simulink model "sus"  (Simulink 6.5)
settings: Solver=ode45  StartTime=0.0  StopTime=16  RelTol=1e-3
libraries: cdsFilt x266, cdsBitwise x92, cdsEpicsOut x84, cdsEpicsBinIn x56, cdsEpicsIn x20, cdsFiltCtrl x18, cdsMatrix x11, cdsSwitch x7, cdsWD x7, cdsFunctionCall x5, cdsRio1 x4, dac x3
(part 2 of 20)

== system sus/LOCK ==
  note: All Outputs the same
  In5 : Inport
  In6 : Inport  Port=2
  In7 : Inport  Port=3
  In8 : Inport  Port=4
  CODE : cdsFunctionCall/Subsystem  Tag=cdsFunctionCall  Description=|  SystemSampleTime=-1
      | Allows to make a call to external C function from the front-end code.                                            
      | User needs to use a Mux and a Demux to proved N number of inputs and M number of outputs to an external function.
      | Function "Foo()" code needs to be put in a file Foo.c in advLigo/src/fe/<model> directory.
      settings: AttributesFormatString=%<Tag>
  DIG4 : cdsFilt/Subsystem  Tag=cdsFilt  Description=|  SystemSampleTime=-1
      | Purpose:                                                                                                                                                                                                                                  
      | Standard CDS IIR filter module.                                                                                                                                                                                                           
      |                                                                                                                                                                                                                                           
      | Operation:                                                                                                                                                                                                                                
      | Consists of 10 second order section IIR filters, plus a ramped gain stage. In FE code, also provides pre-defined test points and excitation channel inputs. The filter coefficients are defined in the LIGO system using the 'foton' tool.
      |                                                                                                                                                                                                                                           
      | Usage:                                                                                                                                                                                                                                    
      | Name the part with the desired filter module name.
      settings: AttributesFormatString=%<Tag>
  Demux : Demux  Outputs=5
  Ground1 : Ground
  Ground7 : Ground
  Mux : Mux  Inputs=6
  OFF : cdsEpicsIn/Subsystem  Tag=cdsEpicsInput  Description=|  SystemSampleTime=-1
      | Purpose:                                                                              
      | Create an EPICS input channel connection to the FE realtime controls.                 
      |                                                                                       
      | Operation:                                                                            
      | Outputs value from an EPICS ai record. Value is floating point with a precision of 3..
      |                                                                                       
      | Usage:                                                                                
      | Name the part with the desired EPICS channel name.
      settings: AttributesFormatString=%<Tag>
  ON : cdsEpicsIn/Subsystem  Tag=cdsEpicsInput  Description=|  SystemSampleTime=-1
      | Purpose:                                                                              
      | Create an EPICS input channel connection to the FE realtime controls.                 
      |                                                                                       
      | Operation:                                                                            
      | Outputs value from an EPICS ai record. Value is floating point with a precision of 3..
      |                                                                                       
      | Usage:                                                                                
      | Name the part with the desired EPICS channel name.
      settings: AttributesFormatString=%<Tag>
  REFL_DC : cdsFilt/Subsystem  Tag=cdsFilt  Description=|  SystemSampleTime=-1
      | Purpose:                                                                                                                                                                                                                                  
      | Standard CDS IIR filter module.                                                                                                                                                                                                           
      |                                                                                                                                                                                                                                           
      | Operation:                                                                                                                                                                                                                                
      | Consists of 10 second order section IIR filters, plus a ramped gain stage. In FE code, also provides pre-defined test points and excitation channel inputs. The filter coefficients are defined in the LIGO system using the 'foton' tool.
      |                                                                                                                                                                                                                                           
      | Usage:                                                                                                                                                                                                                                    
      | Name the part with the desired filter module name.
      settings: AttributesFormatString=%<Tag>
  REFL_I : cdsFilt/Subsystem  Tag=cdsFilt  Description=|  SystemSampleTime=-1
      | Purpose:                                                                                                                                                                                                                                  
      | Standard CDS IIR filter module.                                                                                                                                                                                                           
      |                                                                                                                                                                                                                                           
      | Operation:                                                                                                                                                                                                                                
      | Consists of 10 second order section IIR filters, plus a ramped gain stage. In FE code, also provides pre-defined test points and excitation channel inputs. The filter coefficients are defined in the LIGO system using the 'foton' tool.
      |                                                                                                                                                                                                                                           
      | Usage:                                                                                                                                                                                                                                    
      | Name the part with the desired filter module name.
      settings: AttributesFormatString=%<Tag>
  TRAN_DC : cdsFilt/Subsystem  Tag=cdsFilt  Description=|  SystemSampleTime=-1
      | Purpose:                                                                                                                                                                                                                                  
      | Standard CDS IIR filter module.                                                                                                                                                                                                           
      |                                                                                                                                                                                                                                           
      | Operation:                                                                                                                                                                                                                                
      | Consists of 10 second order section IIR filters, plus a ramped gain stage. In FE code, also provides pre-defined test points and excitation channel inputs. The filter coefficients are defined in the LIGO system using the 'foton' tool.
      |                                                                                                                                                                                                                                           
      | Usage:                                                                                                                                                                                                                                    
      | Name the part with the desired filter module name.
      settings: AttributesFormatString=%<Tag>
  Out1 : Outport
  Out2 : Outport  Port=2
  Out3 : Outport  Port=3
  Out4 : Outport  Port=4
  Out5 : Outport  Port=5
  wires:
  CODE/1 -> Demux/1
  Mux/1 -> CODE/1
  Demux/1 -> Out1/1
  Demux/2 -> Out2/1
  Demux/3 -> Out3/1
  Demux/4 -> Out4/1
  Demux/5 -> Out5/1
  In5/1 -> REFL_I/1
  REFL_I/1 -> Mux/1
  TRAN_DC/1 -> Mux/2
  In6/1 -> TRAN_DC/1
  In7/1 -> REFL_DC/1
  REFL_DC/1 -> Mux/3
  In8/1 -> DIG4/1
  DIG4/1 -> Mux/4
  ON/1 -> Mux/5
  OFF/1 -> Mux/6
  Ground7/1 -> ON/1
  Ground1/1 -> OFF/1

== system sus/MON_M0 ==
  NoiseF1 : Inport  OutDataType=fixdt(1,16,0)  OutScaling=[]
  VoltF1 : Inport  Port=2  OutDataType=fixdt(1,16,0)  OutScaling=[]
  FastF1 : Inport  Port=3  OutDataType=fixdt(1,16,0)  OutScaling=[]
  SlowF1 : Inport  Port=4  OutDataType=fixdt(1,16,0)  OutScaling=[]
  NoiseF2 : Inport  Port=5  OutDataType=fixdt(1,16,0)  OutScaling=[]
  VoltF2 : Inport  Port=6  OutDataType=fixdt(1,16,0)  OutScaling=[]
  FastF2 : Inport  Port=7  OutDataType=fixdt(1,16,0)  OutScaling=[]
  SlowF2 : Inport  Port=8  OutDataType=fixdt(1,16,0)  OutScaling=[]
  NoiseF3 : Inport  Port=9  OutDataType=fixdt(1,16,0)  OutScaling=[]
  VoltF3 : Inport  Port=10  OutDataType=fixdt(1,16,0)  OutScaling=[]
  FastF3 : Inport  Port=11  OutDataType=fixdt(1,16,0)  OutScaling=[]
  SlowF3 : Inport  Port=12  OutDataType=fixdt(1,16,0)  OutScaling=[]
  NoiseLeft : Inport  Port=13  OutDataType=fixdt(1,16,0)  OutScaling=[]
  VoltLeft : Inport  Port=14  OutDataType=fixdt(1,16,0)  OutScaling=[]
  FastLeft : Inport  Port=15  OutDataType=fixdt(1,16,0)  OutScaling=[]
  SlowLeft : Inport  Port=16  OutDataType=fixdt(1,16,0)  OutScaling=[]
  NoiseRight : Inport  Port=17  OutDataType=fixdt(1,16,0)  OutScaling=[]
  VoltRight : Inport  Port=18  OutDataType=fixdt(1,16,0)  OutScaling=[]
  FastRight : Inport  Port=19  OutDataType=fixdt(1,16,0)  OutScaling=[]
  SlowRight : Inport  Port=20  OutDataType=fixdt(1,16,0)  OutScaling=[]
  NoiseSide : Inport  Port=21  OutDataType=fixdt(1,16,0)  OutScaling=[]
  VoltSide : Inport  Port=22  OutDataType=fixdt(1,16,0)  OutScaling=[]
  FastSide : Inport  Port=23  OutDataType=fixdt(1,16,0)  OutScaling=[]
  SlowSide : Inport  Port=24  OutDataType=fixdt(1,16,0)  OutScaling=[]
  FACE1 : Subsystem
  FACE2 : Subsystem
  FACE3 : Subsystem
  LEFT : Subsystem
  RIGHT : Subsystem
  SIDE : Subsystem
  wires:
  NoiseF1/1 -> FACE1/1(Noise)
  VoltF1/1 -> FACE1/2(Volt)
  FastF1/1 -> FACE1/3(Fast I)
  SlowF1/1 -> FACE1/4(Slow I)
  NoiseF2/1 -> FACE2/1(Noise)
  VoltF2/1 -> FACE2/2(Volt)
  FastF2/1 -> FACE2/3(Fast I)
  SlowF2/1 -> FACE2/4(Slow I)
  NoiseF3/1 -> FACE3/1(Noise)
  VoltF3/1 -> FACE3/2(Volt)
  FastF3/1 -> FACE3/3(Fast I)
  SlowF3/1 -> FACE3/4(Slow I)
  NoiseLeft/1 -> LEFT/1(Noise)
  VoltLeft/1 -> LEFT/2(Volt)
  FastLeft/1 -> LEFT/3(Fast I)
  SlowLeft/1 -> LEFT/4(Slow I)
  NoiseRight/1 -> RIGHT/1(Noise)
  VoltRight/1 -> RIGHT/2(Volt)
  FastRight/1 -> RIGHT/3(Fast I)
  SlowRight/1 -> RIGHT/4(Slow I)
  NoiseSide/1 -> SIDE/1(Noise)
  VoltSide/1 -> SIDE/2(Volt)
  FastSide/1 -> SIDE/3(Fast I)
  SlowSide/1 -> SIDE/4(Slow I)

== system sus/MON_PEN ==
  NoiseUL : Inport  OutDataType=fixdt(1,16,0)  OutScaling=[]
  VoltUL : Inport  Port=2  OutDataType=fixdt(1,16,0)  OutScaling=[]
  FastUL : Inport  Port=3  OutDataType=fixdt(1,16,0)  OutScaling=[]
  SlowUL : Inport  Port=4  OutDataType=fixdt(1,16,0)  OutScaling=[]
  NoiseLL : Inport  Port=5  OutDataType=fixdt(1,16,0)  OutScaling=[]
  VoltLL : Inport  Port=6  OutDataType=fixdt(1,16,0)  OutScaling=[]
  FastLL : Inport  Port=7  OutDataType=fixdt(1,16,0)  OutScaling=[]
  SlowLL : Inport  Port=8  OutDataType=fixdt(1,16,0)  OutScaling=[]
  NoiseUR : Inport  Port=9  OutDataType=fixdt(1,16,0)  OutScaling=[]
  VoltUR : Inport  Port=10  OutDataType=fixdt(1,16,0)  OutScaling=[]
  FastUR : Inport  Port=11  OutDataType=fixdt(1,16,0)  OutScaling=[]
  SlowUR : Inport  Port=12  OutDataType=fixdt(1,16,0)  OutScaling=[]
  NoiseLR : Inport  Port=13  OutDataType=fixdt(1,16,0)  OutScaling=[]
  VoltLR : Inport  Port=14  OutDataType=fixdt(1,16,0)  OutScaling=[]
  FastLR : Inport  Port=15  OutDataType=fixdt(1,16,0)  OutScaling=[]
  SlowLR : Inport  Port=16  OutDataType=fixdt(1,16,0)  OutScaling=[]
  LL : Subsystem
  LR : Subsystem
  UL : Subsystem
  UR : Subsystem
  wires:
  NoiseUL/1 -> UL/1(Noise)
  VoltUL/1 -> UL/2(Volt)
  FastUL/1 -> UL/3(Fast I)
  SlowUL/1 -> UL/4(Slow I)
  NoiseLL/1 -> LL/1(Noise)
  VoltLL/1 -> LL/2(Volt)
  FastLL/1 -> LL/3(Fast I)
  SlowLL/1 -> LL/4(Slow I)
  NoiseUR/1 -> UR/1(Noise)
  VoltUR/1 -> UR/2(Volt)
  FastUR/1 -> UR/3(Fast I)
  SlowUR/1 -> UR/4(Slow I)
  NoiseLR/1 -> LR/1(Noise)
  VoltLR/1 -> LR/2(Volt)
  FastLR/1 -> LR/3(Fast I)
  SlowLR/1 -> LR/4(Slow I)

== system sus/MON_R0 ==
  NoiseF1 : Inport  OutDataType=fixdt(1,16,0)  OutScaling=[]
  VoltF1 : Inport  Port=2  OutDataType=fixdt(1,16,0)  OutScaling=[]
  FastF1 : Inport  Port=3  OutDataType=fixdt(1,16,0)  OutScaling=[]
  SlowF1 : Inport  Port=4  OutDataType=fixdt(1,16,0)  OutScaling=[]
  NoiseF2 : Inport  Port=5  OutDataType=fixdt(1,16,0)  OutScaling=[]
  VoltF2 : Inport  Port=6  OutDataType=fixdt(1,16,0)  OutScaling=[]
  FastF2 : Inport  Port=7  OutDataType=fixdt(1,16,0)  OutScaling=[]
  SlowF2 : Inport  Port=8  OutDataType=fixdt(1,16,0)  OutScaling=[]
  NoiseF3 : Inport  Port=9  OutDataType=fixdt(1,16,0)  OutScaling=[]
  VoltF3 : Inport  Port=10  OutDataType=fixdt(1,16,0)  OutScaling=[]
  FastF3 : Inport  Port=11  OutDataType=fixdt(1,16,0)  OutScaling=[]
  SlowF3 : Inport  Port=12  OutDataType=fixdt(1,16,0)  OutScaling=[]
  NoiseLeft : Inport  Port=13  OutDataType=fixdt(1,16,0)  OutScaling=[]
  VoltLeft : Inport  Port=14  OutDataType=fixdt(1,16,0)  OutScaling=[]
  FastLeft : Inport  Port=15  OutDataType=fixdt(1,16,0)  OutScaling=[]
  SlowLeft : Inport  Port=16  OutDataType=fixdt(1,16,0)  OutScaling=[]
  NoiseRight : Inport  Port=17  OutDataType=fixdt(1,16,0)  OutScaling=[]
  VoltRight : Inport  Port=18  OutDataType=fixdt(1,16,0)  OutScaling=[]
  FastRight : Inport  Port=19  OutDataType=fixdt(1,16,0)  OutScaling=[]
  SlowRight : Inport  Port=20  OutDataType=fixdt(1,16,0)  OutScaling=[]
  NoiseSide : Inport  Port=21  OutDataType=fixdt(1,16,0)  OutScaling=[]
  VoltSide : Inport  Port=22  OutDataType=fixdt(1,16,0)  OutScaling=[]
  FastSide : Inport  Port=23  OutDataType=fixdt(1,16,0)  OutScaling=[]
  SlowSide : Inport  Port=24  OutDataType=fixdt(1,16,0)  OutScaling=[]
  FACE1 : Subsystem
  FACE2 : Subsystem
  FACE3 : Subsystem
  LEFT : Subsystem
  RIGHT : Subsystem
  SIDE : Subsystem
  wires:
  NoiseF1/1 -> FACE1/1(Noise)
  VoltF1/1 -> FACE1/2(Volt)
  FastF1/1 -> FACE1/3(Fast I)
  SlowF1/1 -> FACE1/4(Slow I)
  NoiseF2/1 -> FACE2/1(Noise)
  VoltF2/1 -> FACE2/2(Volt)
  FastF2/1 -> FACE2/3(Fast I)
  SlowF2/1 -> FACE2/4(Slow I)
  NoiseF3/1 -> FACE3/1(Noise)
  VoltF3/1 -> FACE3/2(Volt)
  FastF3/1 -> FACE3/3(Fast I)
  SlowF3/1 -> FACE3/4(Slow I)
  NoiseLeft/1 -> LEFT/1(Noise)
  VoltLeft/1 -> LEFT/2(Volt)
  FastLeft/1 -> LEFT/3(Fast I)
  SlowLeft/1 -> LEFT/4(Slow I)
  NoiseRight/1 -> RIGHT/1(Noise)
  VoltRight/1 -> RIGHT/2(Volt)
  FastRight/1 -> RIGHT/3(Fast I)
  SlowRight/1 -> RIGHT/4(Slow I)
  NoiseSide/1 -> SIDE/1(Noise)
  VoltSide/1 -> SIDE/2(Volt)
  FastSide/1 -> SIDE/3(Fast I)
  SlowSide/1 -> SIDE/4(Slow I)

== system sus/MON_UI ==
  NoiseUL : Inport  OutDataType=fixdt(1,16,0)  OutScaling=[]
  VoltUL : Inport  Port=2  OutDataType=fixdt(1,16,0)  OutScaling=[]
  FastUL : Inport  Port=3  OutDataType=fixdt(1,16,0)  OutScaling=[]
  SlowUL : Inport  Port=4  OutDataType=fixdt(1,16,0)  OutScaling=[]
  NoiseLL : Inport  Port=5  OutDataType=fixdt(1,16,0)  OutScaling=[]
  VoltLL : Inport  Port=6  OutDataType=fixdt(1,16,0)  OutScaling=[]
  FastLL : Inport  Port=7  OutDataType=fixdt(1,16,0)  OutScaling=[]
  SlowLL : Inport  Port=8  OutDataType=fixdt(1,16,0)  OutScaling=[]
  NoiseUR : Inport  Port=9  OutDataType=fixdt(1,16,0)  OutScaling=[]
  VoltUR : Inport  Port=10  OutDataType=fixdt(1,16,0)  OutScaling=[]
  FastUR : Inport  Port=11  OutDataType=fixdt(1,16,0)  OutScaling=[]
  SlowUR : Inport  Port=12  OutDataType=fixdt(1,16,0)  OutScaling=[]
  NoiseLR : Inport  Port=13  OutDataType=fixdt(1,16,0)  OutScaling=[]
  VoltLR : Inport  Port=14  OutDataType=fixdt(1,16,0)  OutScaling=[]
  FastLR : Inport  Port=15  OutDataType=fixdt(1,16,0)  OutScaling=[]
  SlowLR : Inport  Port=16  OutDataType=fixdt(1,16,0)  OutScaling=[]
  LL : Subsystem
  LR : Subsystem
  UL : Subsystem
  UR : Subsystem
  wires:
  NoiseUL/1 -> UL/1(Noise)
  VoltUL/1 -> UL/2(Volt)
  FastUL/1 -> UL/3(Fast I)
  SlowUL/1 -> UL/4(Slow I)
  NoiseLL/1 -> LL/1(Noise)
  VoltLL/1 -> LL/2(Volt)
  FastLL/1 -> LL/3(Fast I)
  SlowLL/1 -> LL/4(Slow I)
  NoiseUR/1 -> UR/1(Noise)
  VoltUR/1 -> UR/2(Volt)
  FastUR/1 -> UR/3(Fast I)
  SlowUR/1 -> UR/4(Slow I)
  NoiseLR/1 -> LR/1(Noise)
  VoltLR/1 -> LR/2(Volt)
  FastLR/1 -> LR/3(Fast I)
  SlowLR/1 -> LR/4(Slow I)

== system sus/Q1 ==
  In1 : Inport
  In2 : Inport  Port=2
  In3 : Inport  Port=3
  In4 : Inport  Port=4
  In5 : Inport  Port=5
  In6 : Inport  Port=6
  In7 : Inport  Port=7
  In8 : Inport  Port=8
  In9 : Inport  Port=9
  In10 : Inport  Port=10
  In11 : Inport  Port=11
  In12 : Inport  Port=12
  In13 : Inport  Port=13
  In14 : Inport  Port=14
  In15 : Inport  Port=15
  In16 : Inport  Port=16
  In17 : Inport  Port=17
  In18 : Inport  Port=18
  In19 : Inport  Port=19
  In20 : Inport  Port=20
  OpLevSUM : Inport  Port=21
  OpLevPIT : Inport  Port=22
  OpLevYAW : Inport  Port=23
  POS1 : Inport  Port=24
  POS2 : Inport  Port=25
  POS3 : Inport  Port=26
  ESD : Subsystem
  M0 : Subsystem
  OPLEV : Subsystem
  PEN : Subsystem
  R0 : Subsystem
  SEI_BSC_ACT_SW1 : cdsEpicsOut/Subsystem  Tag=cdsEpicsOutput  Description=|  SystemSampleTime=-1
      | Purpose:                                          
      | Output a FE signal to an EPICS channel.           
      |                                                   
      | Operation:                                        
      | Takes input value and passes it to EPICS record.  
      |                                                   
      | Usage:                                            
      | Name the part with the desired EPICS rrecord name.
      settings: AttributesFormatString=%<Tag>
  SEI_BSC_ACT_SW2 : cdsEpicsOut/Subsystem  Tag=cdsEpicsOutput  Description=|  SystemSampleTime=-1
      | Purpose:                                          
      | Output a FE signal to an EPICS channel.           
      |                                                   
      | Operation:                                        
      | Takes input value and passes it to EPICS record.  
      |                                                   
      | Usage:                                            
      | Name the part with the desired EPICS rrecord name.
      settings: AttributesFormatString=%<Tag>
  SUS_WD_SUM : Logic  Inputs=10  AllPortsSameDT=off  OutDataTypeMode=Boolean
  UI : Subsystem
  M0Face1 : Outport
  M0Face2 : Outport  Port=2
  M0Face3 : Outport  Port=3
  M0Left : Outport  Port=4
  M0Right : Outport  Port=5
  M0Side : Outport  Port=6
  R0Face1 : Outport  Port=7
  R0Face2 : Outport  Port=8
  R0Face3 : Outport  Port=9
  R0Left : Outport  Port=10
  R0Right : Outport  Port=11
  R0Side : Outport  Port=12
  UIUL : Outport  Port=13
  UILL : Outport  Port=14
  UIUR : Outport  Port=15
  UILR : Outport  Port=16
  PenUL : Outport  Port=17
  PenLL : Outport  Port=18
  PenUR : Outport  Port=19
  PenLR : Outport  Port=20
  ESDBias : Outport  Port=21
  ESDQ1 : Outport  Port=22
  ESDQ2 : Outport  Port=23
  ESDQ3 : Outport  Port=24
  ESDQ4 : Outport  Port=25
  wires:
  M0/1(Face1Out) -> M0Face1/1
  M0/2(Face2Out) -> M0Face2/1
  M0/3(Face3Out) -> M0Face3/1
  M0/4(LeftOut) -> M0Left/1
  M0/5(RightOut) -> M0Right/1
  M0/6(SideOut) -> M0Side/1
  R0/1(Face1Out) -> R0Face1/1
  R0/2(Face2Out) -> R0Face2/1
  R0/3(Face3Out) -> R0Face3/1
  R0/4(LeftOut) -> R0Left/1
  R0/6(SideOut) -> R0Side/1
  UI/1(UL) -> UIUL/1
  UI/2(LL) -> UILL/1
  UI/3(UR) -> UIUR/1
  UI/4(LR) -> UILR/1
  R0/5(RightOut) -> R0Right/1
  PEN/1(UR_Out) -> PenUL/1
  PEN/2(UL_Out) -> PenLL/1
  PEN/3(LL_Out) -> PenUR/1
  PEN/4(LR_Out) -> PenLR/1
  M0/7(WD_OUT) -> SUS_WD_SUM/3
  R0/7(WD_OUT) -> SUS_WD_SUM/4
  UI/5(WD_OUT) -> SUS_WD_SUM/5
  PEN/5(WD_OUT) -> SUS_WD_SUM/6
  In1/1 -> M0/1(In1)
  In2/1 -> M0/2(In2)
  In3/1 -> M0/3(In3)
  In4/1 -> M0/4(In4)
  In5/1 -> M0/5(In5)
  In6/1 -> M0/6(In6)
  In7/1 -> R0/1(In1)
  In8/1 -> R0/2(In2)
  In9/1 -> R0/3(In3)
  In10/1 -> R0/4(In4)
  In11/1 -> R0/5(In5)
  In12/1 -> R0/6(In6)
  In13/1 -> UI/1(In1)
  In14/1 -> UI/2(In2)
  In15/1 -> UI/3(In3)
  In16/1 -> UI/4(In4)
  In17/1 -> PEN/1(UR_In)
  In18/1 -> PEN/2(UL_In)
  In19/1 -> PEN/3(LL_In)
  In20/1 -> PEN/4(LR_In)
  OpLevSUM/1 -> OPLEV/1(InSUM)
  OpLevPIT/1 -> OPLEV/2(InPIT)
  OpLevYAW/1 -> OPLEV/3(InYAW)
  OPLEV/1(OutPIT) -> ESD/2(In2), UI/6(In6), PEN/6(In6)
  OPLEV/2(OutYAW) -> ESD/3(In3), UI/7(In7), PEN/7(In7)
  ESD/1(Out1) -> ESDBias/1
  ESD/2(Out2) -> ESDQ1/1
  ESD/3(Out3) -> ESDQ2/1
  ESD/4(Out4) -> ESDQ3/1
  ESD/5(Out5) -> ESDQ4/1
  POS1/1 -> UI/5(In5), M0/7(LSC_In)
  POS3/1 -> ESD/1(In1)
  POS2/1 -> PEN/5(In5)
  M0/8(Quad_rm_wd) -> SUS_WD_SUM/1
  SUS_WD_SUM/1 -> SEI_BSC_ACT_SW1/1, SEI_BSC_ACT_SW2/1
  R0/8(Quad_rm_wd) -> SUS_WD_SUM/2
  M0/9(WD_SW_Status) -> SUS_WD_SUM/7
  R0/9(WD_SW_Status) -> SUS_WD_SUM/8
  UI/6(WD_SW_Status) -> SUS_WD_SUM/9
  PEN/6(WD_SW_Status) -> SUS_WD_SUM/10
